simulink model "model_examples"  (Simulink 7.5)
settings: Solver=ode45  StartTime=0.0  StopTime=10.0  RelTol=1e-3
undefined symbols (not defined in the file): I, K
settings Model: Creator=jporter  LastModifiedBy=jporter

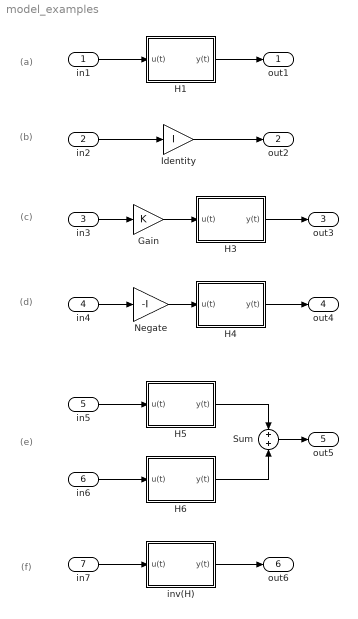
== system model_examples ==
  note: (a)
  note: (c)
  note: (b)
  note: (d)
  note: (e)
  note: (f)
  in1 : Inport  OutDataType=fixdt(1, 16)  OutScaling=2^0
  in2 : Inport  Port=2  OutDataType=fixdt(1, 16)  OutScaling=2^0
  in3 : Inport  Port=3  OutDataType=fixdt(1, 16)  OutScaling=2^0
  in4 : Inport  Port=4  OutDataType=fixdt(1, 16)  OutScaling=2^0
  in5 : Inport  Port=5  OutDataType=fixdt(1, 16)  OutScaling=2^0
  in6 : Inport  Port=6  OutDataType=fixdt(1, 16)  OutScaling=2^0
  in7 : Inport  Port=7  OutDataType=fixdt(1, 16)  OutScaling=2^0
  Gain : Gain  Gain=K  ParameterDataType=fixdt(1, 16)  ParameterScaling=2^0  OutDataType=fixdt(1, 16)  OutScaling=2^0
  H1 : Subsystem
  H3 : Subsystem
  H4 : Subsystem
  H5 : Subsystem
  H6 : Subsystem
  Identity : Gain  Gain=I  ParameterDataType=fixdt(1, 16)  ParameterScaling=2^0  OutDataType=fixdt(1, 16)  OutScaling=2^0
  Negate : Gain  Gain=-I  ParameterDataType=fixdt(1, 16)  ParameterScaling=2^0  OutDataType=fixdt(1, 16)  OutScaling=2^0
  Sum : Sum  Inputs=+|+  OutDataType=fixdt(1, 16)  OutScaling=2^0
  inv(H) : Subsystem
  out1 : Outport  OutDataType=fixdt(1, 16)  OutScaling=2^0
  out2 : Outport  Port=2  OutDataType=fixdt(1, 16)  OutScaling=2^0
  out3 : Outport  Port=3  OutDataType=fixdt(1, 16)  OutScaling=2^0
  out4 : Outport  Port=4  OutDataType=fixdt(1, 16)  OutScaling=2^0
  out5 : Outport  Port=5  OutDataType=fixdt(1, 16)  OutScaling=2^0
  out6 : Outport  Port=6  OutDataType=fixdt(1, 16)  OutScaling=2^0
  wires:
  in1/1 -> H1/1(u(t))
  H1/1(y(t)) -> out1/1
  in3/1 -> Gain/1
  H3/1(y(t)) -> out3/1
  Gain/1 -> H3/1(u(t))
  in2/1 -> Identity/1
  Identity/1 -> out2/1
  in4/1 -> Negate/1
  H4/1(y(t)) -> out4/1
  Negate/1 -> H4/1(u(t))
  in5/1 -> H5/1(u(t))
  in6/1 -> H6/1(u(t))
  H5/1(y(t)) -> Sum/1
  Sum/1 -> out5/1
  H6/1(y(t)) -> Sum/2
  in7/1 -> inv(H)/1(u(t))
  inv(H)/1(y(t)) -> out6/1

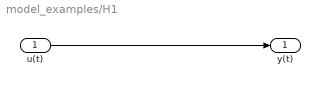
== system model_examples/H1 ==
  u(t) : Inport  OutDataType=fixdt(1, 16)  OutScaling=2^0
  y(t) : Outport  OutDataType=fixdt(1, 16)  OutScaling=2^0
  wires:
  u(t)/1 -> y(t)/1

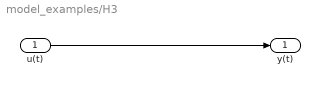
== system model_examples/H3 ==
  u(t) : Inport  OutDataType=fixdt(1, 16)  OutScaling=2^0
  y(t) : Outport  OutDataType=fixdt(1, 16)  OutScaling=2^0
  wires:
  u(t)/1 -> y(t)/1

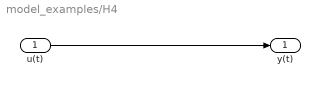
== system model_examples/H4 ==
  u(t) : Inport  OutDataType=fixdt(1, 16)  OutScaling=2^0
  y(t) : Outport  OutDataType=fixdt(1, 16)  OutScaling=2^0
  wires:
  u(t)/1 -> y(t)/1

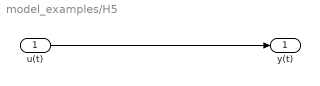
== system model_examples/H5 ==
  u(t) : Inport  OutDataType=fixdt(1, 16)  OutScaling=2^0
  y(t) : Outport  OutDataType=fixdt(1, 16)  OutScaling=2^0
  wires:
  u(t)/1 -> y(t)/1

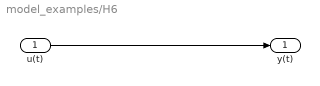
== system model_examples/H6 ==
  u(t) : Inport  OutDataType=fixdt(1, 16)  OutScaling=2^0
  y(t) : Outport  OutDataType=fixdt(1, 16)  OutScaling=2^0
  wires:
  u(t)/1 -> y(t)/1

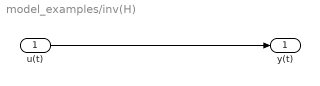
== system model_examples/inv(H) ==
  u(t) : Inport  OutDataType=fixdt(1, 16)  OutScaling=2^0
  y(t) : Outport  OutDataType=fixdt(1, 16)  OutScaling=2^0
  wires:
  u(t)/1 -> y(t)/1
